simulink library "ddm"  (R2021b)
settings: Solver=VariableStepAuto  StartTime=0.0  StopTime=10.0  RelTol=1e-3
undefined symbols (not defined in the file): ADDM_FrTMTqDev_X_Nm, ADDM_RrTMTqDev_X_Nm, ENUM_ADASACCSTA_ERROR, ENUM_ADASACCSTA_OFF, ENUM_ADASACCSTA_STANDBY, ENUM_ALLOWMOV_ALLOWREADY, ENUM_APS, ENUM_BRKSTA_ERROR, ENUM_BRKSTA_OFF, ENUM_BRKSTA_ON, ENUM_BRKSW_INVALID, ENUM_BRKSW_OFF, ENUM_BRKSW_ON, ENUM_CHGPREACTERRSTA_OBCPRE, ENUM_DCDCFAULTSTA_ANYFAULTLV1, ENUM_DCDCFAULTSTA_ANYFAULTLV2, ENUM_DRIVETRAIN_AWD, ENUM_DRIVETRAIN_FWD, ENUM_DRIVETRAIN_RWD, ENUM_EDUDRTSTA_NORMAL, ENUM_EPBERROR_FAILED, ENUM_EPBSTA_APPLIED, ENUM_EPBSTA_RELEASED, ENUM_ESCAPSSta_APSUNAVAILABLE, ENUM_GEARACTUALPOSN_INVALID, ENUM_GEARACTUALPOSN_P, ENUM_HVBATTREADYPRE_READY, ENUM_HWRESETSTA_HWRESETING, ENUM_MCUWARN_LV0, ENUM_MCUWARN_LV1, ENUM_MCUWARN_LV2, ENUM_MCUWARN_LV3, ENUM_MCUWARN_NOERROR, ENUM_OBCFAULTSTA_ANYFAULT, ENUM_PAS_R2F2, ENUM_PDFAULT_BATTPDFAIL, ENUM_PDFAULT_DCDCDISABLE, ENUM_PDFAULT_MCUDISABLE, ENUM_PDFAULT_MCUDISCHRG, ENUM_POWERSTA_OFF, ENUM_POWERSTA_ON, ENUM_POWERSTA_READY, ENUM_POWERSTA_STANDBY, ENUM_PRESSINDI_LOW, ENUM_PUFAULT_BATTUPFAIL, ENUM_PUFAULT_DCDCENABLEFAIL, ENUM_PUFAULT_PRECHRGCHKFAIL, ENUM_PUFAULT_SAFETYCHKFAIL, ENUM_PWRSTASW_OFF, ENUM_PWRSTASW_OFFA, ENUM_PWRSTASW_OFFCHVCHRG, ENUM_PWRSTASW_OFFCLVCHRG, ENUM_PWRSTASW_ON, ENUM_PWRSTASW_ONHVCHRG, ENUM_PWRSTASW_READY, ENUM_PWRSTASW_STANDBY, ENUM_RAPSErrWarnSta_NORMAL, ENUM_RAPSErrWarnSta_RAPSERRLV1, ENUM_SHIFTCOMMAND_P, ENUM_SHIFTERERRSTA_PBUTTONFAILURE ... (+471)
libraries: hcu_lib x540, simulink x3
(part 12 of 26)

== system ddm/DDM/DDM/TPM/RRBatwarn ==
  note: Diagnostics and Fault Handling
  note: Release Condition After Decision
  note: Test Pass Criteria
  note: Test Detection Criteria
  task_time_s : Inport
  VPMM_PowerSta_enum : Inport  Port=2
  DTC_clear_request : Inport  Port=3
  VTPM_RRBatwarn_flg : Inport  Port=4
  Constant : Constant  Value=KDDM_RRBatwarnDTC_cnt
  Constant1 : Constant  Value=KDDM_RRBatwarnDTC_cnt
  Constant10 : Constant  Value=ENUM_POWERSTA_OFF
  Constant11 : Constant  Value=KDDM_RRBatwarnPassSW_flg
  Constant12 : Constant  Value=FALSE
  Constant13 : Constant  Value=KDDM_RRBatwarnCFSSW_flg
  Constant14 : Constant  Value=KDDM_RRBatwarnDFSSW_flg
  Constant15 : Constant  Value=KDDM_RRBatwarnDetTO_s
  Constant16 : Constant  Value=KDDM_RRBatwarnDetTO_s
  Constant2 : Constant  Value=ENUM_POWERSTA_READY
  Constant24 : Constant  Value=TRUE
  Constant25 : Constant  Value=FALSE
  Constant3 : Constant  Value=ENUM_POWERSTA_ON
  Constant4 : Constant  Value=FALSE
  Constant46 : Constant  Value=KDDM_RRBatwarnDetSW_flg
  Constant5 : Constant  Value=ENUM_POWERSTA_READY
  Constant6 : Constant  Value=KDDM_RRBatwarnDetTO_s
  Constant7 : Constant  Value=ENUM_POWERSTA_ON
  Constant8 : Constant  Value=TRUE
  DTC_Couter : hcu_lib/Basic_Blocks/DTC_Couter
  DTC_Info : hcu_lib/Basic_Blocks/DTC_Info
  Data Type Conversion1 : DataTypeConversion  OutDataTypeStr=uint8
  Equal{1..5} (5 alike) : RelationalOperator  Operator===  OutDataTypeStr=boolean  RndMeth=Simplest
  Equal6 : RelationalOperator  OutDataTypeStr=boolean  RndMeth=Simplest
  Logical Operator1 : Logic  Operator=OR  AllPortsSameDT=off  OutDataTypeStr=boolean
  Logical Operator12 : Logic  AllPortsSameDT=off  OutDataTypeStr=boolean
  Logical Operator15 : Logic  AllPortsSameDT=off  OutDataTypeStr=boolean
  Logical Operator18 : Logic  AllPortsSameDT=off  OutDataTypeStr=boolean
  Logical Operator19 : Logic  Inputs=3  AllPortsSameDT=off  OutDataTypeStr=boolean
  Logical Operator2 : Logic  Operator=NOT  AllPortsSameDT=off  OutDataTypeStr=boolean
  Logical Operator3 : Logic  Operator=OR  Inputs=3  AllPortsSameDT=off  OutDataTypeStr=boolean
  Logical Operator4 : Logic  Operator=OR  AllPortsSameDT=off  OutDataTypeStr=boolean
  Logical Operator5 : Logic  Operator=OR  Inputs=2.  AllPortsSameDT=off  OutDataTypeStr=boolean
  Logical Operator6 : Logic  Operator=NOT  AllPortsSameDT=off  OutDataTypeStr=boolean
  Logical Operator7 : Logic  Operator=OR  Inputs=2.  AllPortsSameDT=off  OutDataTypeStr=boolean
  Logical Operator8 : Logic  Operator=OR  AllPortsSameDT=off  OutDataTypeStr=boolean
  Relay : Relay  OnSwitchValue=ONE_INT  OffSwitchValue=ZERO_INT
  SR_Latch1 : Subsystem  mask(SR_Latch){}
      mask help: SR latch function.
  SR_Latch3 : hcu_lib/Basic_Blocks/SR_Latch
  SR_Latch4 : hcu_lib/Basic_Blocks/SR_Latch
  Switch{2..4,6} (4 alike) : Switch  Criteria=u2 ~= 0
  Test Detection Criteria : hcu_lib/Basic_Blocks/Test Detection Criteria
  Timer1 : hcu_lib/Basic_Blocks/Timer
  VDDM_RRBatwarnDTC_raw32 : Outport
  wires:
  Switch6/1 -> Test Detection Criteria/1
  Constant12/1 -> Switch6/1
  [DTC_clear_request] -> Switch6/2
  Switch3/1 -> [VDDM_RRBatwarnChk_flg], Switch6/3
  VTPM_RRBatwarn_flg/1 -> [VTPM_RRBatwarn_flg]
  [VTPM_RRBatwarn_flg] -> Switch4/1
  Logical Operator4/1 -> Switch4/2
  Equal3/1 -> Logical Operator4/1
  [VPMM_PowerSta_enum] -> Equal2/1
  Constant7/1 -> Equal3/2
  Constant5/1 -> Equal2/2
  Constant8/1 -> Switch4/3
  Equal2/1 -> Logical Operator4/2
  [VPMM_PowerSta_enum] -> Equal3/1
  [VTPM_RRBatwarn_flg] -> Switch3/1
  [task_time_s] -> Test Detection Criteria/2
  Constant/1 -> Test Detection Criteria/3
  Constant6/1 -> Test Detection Criteria/4
  [VPMM_PowerSta_enum] -> Equal5/1
  Equal1/1 -> Logical Operator1/2
  Equal5/1 -> Logical Operator1/1
  Logical Operator1/1 -> Switch3/2
  Constant3/1 -> Equal5/2
  Constant2/1 -> Equal1/2
  Constant4/1 -> Switch3/3
  [VPMM_PowerSta_enum] -> Equal1/1
  [DTC_clear_request] -> DTC_Info/4
  [VDDM_RRBatwarnPass_flg] -> DTC_Info/2
  [VDDM_RRBatwarnDet_flg] -> DTC_Info/1
  Test Detection Criteria/1 -> [VDDM_RRBatwarnDet_flg]  "VDDM_RRBatwarnDet_flg"
  DTC_Info/1 -> VDDM_RRBatwarnDTC_raw32/1  "VDDM_RRBatwarnDTC_raw32"
  [VDDM_RRBatwarnCFS_flg] -> DTC_Info/3
  [VPMM_PowerSta_enum] -> Equal4/1
  DTC_clear_request/1 -> [DTC_clear_request]
  [VDDM_RRBatwarnCFSRls_flg] -> Logical Operator3/3
  Logical Operator18/1 -> [VDDM_RRBatwarnCFS_flg]
  Constant14/1 -> Logical Operator12/1
  SR_Latch3/1 -> Logical Operator12/2
  Constant13/1 -> Logical Operator18/2
  Logical Operator12/1 -> [VDDM_RRBatwarnDFS_flg]
  SR_Latch4/1 -> Logical Operator18/1
  [VDDM_RRBatwarnCFSRls_flg] -> Logical Operator5/1
  [VDDM_RRBatwarnPass_flg] -> Logical Operator3/2
  DTC_Couter/1 -> SR_Latch4/1
  Data Type Conversion1/1 -> [VDDM_RRBatwarnDTC_cnt]  "VDDM_RRBatwarnDTC_cnt"
  Constant46/1 -> Logical Operator19/2
  Logical Operator19/1 -> DTC_Couter/1
  Constant11/1 -> Logical Operator15/2
  Logical Operator15/1 -> DTC_Couter/2
  Constant1/1 -> DTC_Couter/3
  DTC_Couter/2 -> Data Type Conversion1/1
  Relay/1 -> SR_Latch3/1
  [VDDM_RRBatwarnDet_flg] -> Logical Operator19/1
  Logical Operator3/1 -> Logical Operator15/1
  [VDDM_RRBatwarnCFS_flg] -> Logical Operator7/1
  [VDDM_RRBatwarnDTC_cnt] -> Relay/1
  Equal4/1 -> Logical Operator8/1
  Constant10/1 -> Equal4/2
  Constant24/1 -> Switch2/1
  [DTC_clear_request] -> Logical Operator8/2
  Switch2/1 -> [VDDM_RRBatwarnCFSRls_flg]
  Constant25/1 -> Switch2/3
  Logical Operator8/1 -> Switch2/2
  VPMM_PowerSta_enum/1 -> [VPMM_PowerSta_enum]
  task_time_s/1 -> [task_time_s]
  Switch4/1 -> Timer1/2, Logical Operator6/1
  Equal6/1 -> SR_Latch1/1(set)
  [VDDM_RRBatwarnChk_flg] -> SR_Latch1/2(reset)
  Timer1/1 -> Equal6/1
  Constant16/1 -> Equal6/2
  SR_Latch1/1(latched) -> [VDDM_RRBatwarnPass_flg]
  [task_time_s] -> Timer1/3
  Logical Operator6/1 -> Timer1/1
  Constant15/1 -> Timer1/4
  Logical Operator2/1 -> Logical Operator19/3
  [DTC_clear_request] -> Logical Operator3/1, Logical Operator2/1
  Logical Operator5/1 -> SR_Latch4/2
  [DTC_clear_request] -> Logical Operator5/2
  Logical Operator7/1 -> SR_Latch3/2
  [DTC_clear_request] -> Logical Operator7/2

== system ddm/DDM/DDM/TPM/RRPressureLow ==
  note: Test Detection Criteria
  note: Test Pass Criteria
  note: Release Condition After Decision
  note: Diagnostics and Fault Handling
  task_time_s : Inport
  VPMM_PowerSta_enum : Inport  Port=2
  DTC_clear_request : Inport  Port=3
  VTPM_RRPressIndi_enum : Inport  Port=4
  Constant : Constant  Value=KDDM_RRPressIndiDTC_cnt
  Constant1 : Constant  Value=KDDM_RRPressIndiDTC_cnt
  Constant10 : Constant  Value=ENUM_POWERSTA_OFF
  Constant11 : Constant  Value=KDDM_RRPressIndiPassSW_flg
  Constant12 : Constant  Value=FALSE
  Constant13 : Constant  Value=KDDM_RRPressIndiCFSSW_flg
  Constant14 : Constant  Value=KDDM_RRPressIndiDFSSW_flg
  Constant15 : Constant  Value=KDDM_RRPressIndiPassTO_s
  Constant16 : Constant  Value=ENUM_PRESSINDI_LOW
  Constant17 : Constant  Value=ENUM_PRESSINDI_LOW
  Constant2 : Constant  Value=ENUM_POWERSTA_READY
  Constant24 : Constant  Value=TRUE
  Constant25 : Constant  Value=FALSE
  Constant3 : Constant  Value=ENUM_POWERSTA_ON
  Constant4 : Constant  Value=FALSE
  Constant46 : Constant  Value=KDDM_RRPressIndiDetSW_flg
  Constant5 : Constant  Value=ENUM_POWERSTA_READY
  Constant6 : Constant  Value=KDDM_RRPressIndiDetTO_s
  Constant7 : Constant  Value=ENUM_POWERSTA_ON
  Constant8 : Constant  Value=TRUE
  Constant9 : Constant  Value=KDDM_RRPressIndiPassTO_s
  DTC_Couter : hcu_lib/Basic_Blocks/DTC_Couter
  DTC_Info : hcu_lib/Basic_Blocks/DTC_Info
  Data Type Conversion1 : DataTypeConversion  OutDataTypeStr=uint8
  Equal{1..5,7..8} (7 alike) : RelationalOperator  Operator===  OutDataTypeStr=boolean  RndMeth=Simplest
  Equal6 : RelationalOperator  OutDataTypeStr=boolean  RndMeth=Simplest
  Logical Operator{1,4..5,7..8} (5 alike) : Logic  Operator=OR  AllPortsSameDT=off  OutDataTypeStr=boolean
  Logical Operator12 : Logic  AllPortsSameDT=off  OutDataTypeStr=boolean
  Logical Operator15 : Logic  AllPortsSameDT=off  OutDataTypeStr=boolean
  Logical Operator18 : Logic  AllPortsSameDT=off  OutDataTypeStr=boolean
  Logical Operator19 : Logic  Inputs=3  AllPortsSameDT=off  OutDataTypeStr=boolean
  Logical Operator2 : Logic  Operator=NOT  AllPortsSameDT=off  OutDataTypeStr=boolean
  Logical Operator3 : Logic  Operator=OR  Inputs=3  AllPortsSameDT=off  OutDataTypeStr=boolean
  Logical Operator6 : Logic  Operator=NOT  AllPortsSameDT=off  OutDataTypeStr=boolean
  Relay : Relay  OnSwitchValue=ONE_INT  OffSwitchValue=ZERO_INT
  SR_Latch1 : Subsystem  mask(SR_Latch){}
      mask help: SR latch function.
  SR_Latch3 : hcu_lib/Basic_Blocks/SR_Latch
  SR_Latch4 : hcu_lib/Basic_Blocks/SR_Latch
  Switch{2..4,6} (4 alike) : Switch  Criteria=u2 ~= 0
  Test Detection Criteria : hcu_lib/Basic_Blocks/Test Detection Criteria
  Timer1 : hcu_lib/Basic_Blocks/Timer
  VDDM_RRPressIndiDTC_raw32 : Outport
  wires:
  [VTPM_RRPressIndi_enum] -> Equal8/1
  Constant17/1 -> Equal8/2
  Equal8/1 -> Switch4/1
  Constant16/1 -> Equal7/2
  Equal7/1 -> Switch3/1
  [VTPM_RRPressIndi_enum] -> Equal7/1
  task_time_s/1 -> [task_time_s]
  VPMM_PowerSta_enum/1 -> [VPMM_PowerSta_enum]
  Logical Operator8/1 -> Switch2/2
  Constant25/1 -> Switch2/3
  Switch2/1 -> [VDDM_RRPressIndiCFSRls_flg]
  [DTC_clear_request] -> Logical Operator8/2
  Constant24/1 -> Switch2/1
  Constant10/1 -> Equal4/2
  Equal4/1 -> Logical Operator8/1
  [VDDM_RRPressIndiDTC_cnt] -> Relay/1
  [VDDM_RRPressIndiCFS_flg] -> Logical Operator7/1
  Logical Operator3/1 -> Logical Operator15/1
  [VDDM_RRPressIndiDet_flg] -> Logical Operator19/1
  Relay/1 -> SR_Latch3/1
  Constant1/1 -> DTC_Couter/3
  Logical Operator15/1 -> DTC_Couter/2
  Constant11/1 -> Logical Operator15/2
  Logical Operator19/1 -> DTC_Couter/1
  Constant46/1 -> Logical Operator19/2
  DTC_Couter/1 -> SR_Latch4/1
  [VDDM_RRPressIndiPass_flg] -> Logical Operator3/2
  [VDDM_RRPressIndiCFSRls_flg] -> Logical Operator5/1
  SR_Latch4/1 -> Logical Operator18/1
  Logical Operator12/1 -> [VDDM_RRPressIndiDFS_flg]
  Constant13/1 -> Logical Operator18/2
  SR_Latch3/1 -> Logical Operator12/2
  Constant14/1 -> Logical Operator12/1
  Logical Operator18/1 -> [VDDM_RRPressIndiCFS_flg]
  [VDDM_RRPressIndiCFSRls_flg] -> Logical Operator3/3
  DTC_clear_request/1 -> [DTC_clear_request]
  [VPMM_PowerSta_enum] -> Equal4/1
  [VDDM_RRPressIndiCFS_flg] -> DTC_Info/3
  DTC_Info/1 -> VDDM_RRPressIndiDTC_raw32/1  "VDDM_RRPressIndiDTC_raw32"
  Test Detection Criteria/1 -> [VDDM_RRPressIndiDet_flg]  "VDDM_RRPressIndiDet_flg"
  [VDDM_RRPressIndiDet_flg] -> DTC_Info/1
  [VDDM_RRPressIndiPass_flg] -> DTC_Info/2
  [DTC_clear_request] -> DTC_Info/4
  [VPMM_PowerSta_enum] -> Equal1/1
  Constant4/1 -> Switch3/3
  Constant5/1 -> Equal1/2
  Constant7/1 -> Equal5/2
  Logical Operator1/1 -> Switch3/2
  Equal5/1 -> Logical Operator1/1
  Equal1/1 -> Logical Operator1/2
  [VPMM_PowerSta_enum] -> Equal5/1
  Constant6/1 -> Test Detection Criteria/4
  Constant/1 -> Test Detection Criteria/3
  [task_time_s] -> Test Detection Criteria/2
  [VPMM_PowerSta_enum] -> Equal3/1
  Equal2/1 -> Logical Operator4/2
  Constant8/1 -> Switch4/3
  Constant2/1 -> Equal2/2
  Constant3/1 -> Equal3/2
  [VPMM_PowerSta_enum] -> Equal2/1
  Equal3/1 -> Logical Operator4/1
  Logical Operator4/1 -> Switch4/2
  VTPM_RRPressIndi_enum/1 -> [VTPM_RRPressIndi_enum]
  Switch3/1 -> [VDDM_RRPressIndiChk_flg], Switch6/3
  [DTC_clear_request] -> Switch6/2
  Constant12/1 -> Switch6/1
  Switch6/1 -> Test Detection Criteria/1
  Switch4/1 -> Logical Operator6/1, Timer1/2
  Equal6/1 -> SR_Latch1/1(set)
  Constant9/1 -> Equal6/2
  SR_Latch1/1(latched) -> [VDDM_RRPressIndiPass_flg]
  [VDDM_RRPressIndiChk_flg] -> SR_Latch1/2(reset)
  [task_time_s] -> Timer1/3
  Timer1/1 -> Equal6/1
  Constant15/1 -> Timer1/4
  Logical Operator6/1 -> Timer1/1
  Data Type Conversion1/1 -> [VDDM_RRPressIndiDTC_cnt]  "VDDM_RRPressIndiDTC_cnt"
  DTC_Couter/2 -> Data Type Conversion1/1
  Logical Operator2/1 -> Logical Operator19/3
  [DTC_clear_request] -> Logical Operator3/1, Logical Operator2/1
  Logical Operator5/1 -> SR_Latch4/2
  [DTC_clear_request] -> Logical Operator5/2
  Logical Operator7/1 -> SR_Latch3/2
  [DTC_clear_request] -> Logical Operator7/2

== system ddm/DDM/DDM/TPM/RRSensorfail ==
  note: Test Detection Criteria
  note: Test Pass Criteria
  note: Release Condition After Decision
  note: Diagnostics and Fault Handling
  task_time_s : Inport
  VPMM_PowerSta_enum : Inport  Port=2
  DTC_clear_request : Inport  Port=3
  VTPM_RRSensorFail_flg : Inport  Port=4
  Constant : Constant  Value=KDDM_RRSensorFailDTC_cnt
  Constant1 : Constant  Value=KDDM_RRSensorFailDTC_cnt
  Constant10 : Constant  Value=ENUM_POWERSTA_OFF
  Constant11 : Constant  Value=KDDM_RRSensorFailPassSW_flg
  Constant12 : Constant  Value=FALSE
  Constant13 : Constant  Value=KDDM_RRSensorFailCFSSW_flg
  Constant14 : Constant  Value=KDDM_RRSensorFailDFSSW_flg
  Constant15 : Constant  Value=KDDM_RRSensorFailPassTO_s
  Constant2 : Constant  Value=ENUM_POWERSTA_READY
  Constant24 : Constant  Value=TRUE
  Constant25 : Constant  Value=FALSE
  Constant3 : Constant  Value=ENUM_POWERSTA_ON
  Constant4 : Constant  Value=FALSE
  Constant46 : Constant  Value=KDDM_RRSensorFailDetSW_flg
  Constant5 : Constant  Value=ENUM_POWERSTA_READY
  Constant6 : Constant  Value=KDDM_RRSensorFailDetTO_s
  Constant7 : Constant  Value=ENUM_POWERSTA_ON
  Constant8 : Constant  Value=TRUE
  Constant9 : Constant  Value=KDDM_RRSensorFailPassTO_s
  DTC_Couter : hcu_lib/Basic_Blocks/DTC_Couter
  DTC_Info : hcu_lib/Basic_Blocks/DTC_Info
  Data Type Conversion1 : DataTypeConversion  OutDataTypeStr=uint8
  Equal{1..5} (5 alike) : RelationalOperator  Operator===  OutDataTypeStr=boolean  RndMeth=Simplest
  Equal6 : RelationalOperator  OutDataTypeStr=boolean  RndMeth=Simplest
  Logical Operator{1..2,4,7..8} (5 alike) : Logic  Operator=OR  AllPortsSameDT=off  OutDataTypeStr=boolean
  Logical Operator12 : Logic  AllPortsSameDT=off  OutDataTypeStr=boolean
  Logical Operator15 : Logic  AllPortsSameDT=off  OutDataTypeStr=boolean
  Logical Operator18 : Logic  AllPortsSameDT=off  OutDataTypeStr=boolean
  Logical Operator19 : Logic  Inputs=3  AllPortsSameDT=off  OutDataTypeStr=boolean
  Logical Operator3 : Logic  Operator=OR  Inputs=3  AllPortsSameDT=off  OutDataTypeStr=boolean
  Logical Operator5 : Logic  Operator=NOT  AllPortsSameDT=off  OutDataTypeStr=boolean
  Logical Operator6 : Logic  Operator=NOT  AllPortsSameDT=off  OutDataTypeStr=boolean
  Relay : Relay  OnSwitchValue=ONE_INT  OffSwitchValue=ZERO_INT
  SR_Latch1 : Subsystem  mask(SR_Latch){}
      mask help: SR latch function.
  SR_Latch3 : hcu_lib/Basic_Blocks/SR_Latch
  SR_Latch4 : hcu_lib/Basic_Blocks/SR_Latch
  Switch{2..4,6} (4 alike) : Switch  Criteria=u2 ~= 0
  Test Detection Criteria : hcu_lib/Basic_Blocks/Test Detection Criteria
  Timer1 : hcu_lib/Basic_Blocks/Timer
  VDDM_RRSensorFailDTC_raw32 : Outport
  wires:
  [VTPM_RRSensorFail_flg] -> Switch4/1
  [VTPM_RRSensorFail_flg] -> Switch3/1
  task_time_s/1 -> [task_time_s]
  VPMM_PowerSta_enum/1 -> [VPMM_PowerSta_enum]
  Logical Operator8/1 -> Switch2/2
  Constant25/1 -> Switch2/3
  Switch2/1 -> [VDDM_RRSensorFailCFSRls_flg]
  [DTC_clear_request] -> Logical Operator8/2
  Constant24/1 -> Switch2/1
  Constant10/1 -> Equal4/2
  Equal4/1 -> Logical Operator8/1
  [VDDM_RRSensorFailDTC_cnt] -> Relay/1
  [VDDM_RRSensorFailCFS_flg] -> Logical Operator7/1
  Logical Operator3/1 -> Logical Operator15/1
  [VDDM_RRSensorFailDet_flg] -> Logical Operator19/1
  Relay/1 -> SR_Latch3/1
  DTC_Couter/2 -> Data Type Conversion1/1
  Constant1/1 -> DTC_Couter/3
  Logical Operator15/1 -> DTC_Couter/2
  Constant11/1 -> Logical Operator15/2
  Logical Operator19/1 -> DTC_Couter/1
  Constant46/1 -> Logical Operator19/2
  Data Type Conversion1/1 -> [VDDM_RRSensorFailDTC_cnt]  "VDDM_RRSensorFailDTC_cnt"
  DTC_Couter/1 -> SR_Latch4/1
  [VDDM_RRSensorFailPass_flg] -> Logical Operator3/2
  [VDDM_RRSensorFailCFSRls_flg] -> Logical Operator2/1
  SR_Latch4/1 -> Logical Operator18/1
  Logical Operator12/1 -> [VDDM_RRSensorFailDFS_flg]
  Constant13/1 -> Logical Operator18/2
  SR_Latch3/1 -> Logical Operator12/2
  Constant14/1 -> Logical Operator12/1
  Logical Operator18/1 -> [VDDM_RRSensorFailCFS_flg]
  [VDDM_RRSensorFailCFSRls_flg] -> Logical Operator3/3
  DTC_clear_request/1 -> [DTC_clear_request]
  [VPMM_PowerSta_enum] -> Equal4/1
  [VDDM_RRSensorFailCFS_flg] -> DTC_Info/3
  DTC_Info/1 -> VDDM_RRSensorFailDTC_raw32/1  "VDDM_RRSensorFailDTC_raw32"
  Test Detection Criteria/1 -> [VDDM_RRSensorFailDet_flg]  "VDDM_RRSensorFailDet_flg"
  [VDDM_RRSensorFailDet_flg] -> DTC_Info/1
  [VDDM_RRSensorFailPass_flg] -> DTC_Info/2
  [DTC_clear_request] -> DTC_Info/4
  [VPMM_PowerSta_enum] -> Equal1/1
  Constant4/1 -> Switch3/3
  Constant5/1 -> Equal1/2
  Constant7/1 -> Equal5/2
  Logical Operator1/1 -> Switch3/2
  Equal5/1 -> Logical Operator1/1
  Equal1/1 -> Logical Operator1/2
  [VPMM_PowerSta_enum] -> Equal5/1
  Constant6/1 -> Test Detection Criteria/4
  Constant/1 -> Test Detection Criteria/3
  [task_time_s] -> Test Detection Criteria/2
  [VPMM_PowerSta_enum] -> Equal3/1
  Equal2/1 -> Logical Operator4/2
  Constant8/1 -> Switch4/3
  Constant2/1 -> Equal2/2
  Constant3/1 -> Equal3/2
  [VPMM_PowerSta_enum] -> Equal2/1
  Equal3/1 -> Logical Operator4/1
  Logical Operator4/1 -> Switch4/2
  VTPM_RRSensorFail_flg/1 -> [VTPM_RRSensorFail_flg]
  Switch3/1 -> [VDDM_RRSensorFailChk_flg], Switch6/3
  [DTC_clear_request] -> Switch6/2
  Constant12/1 -> Switch6/1
  Switch6/1 -> Test Detection Criteria/1
  Switch4/1 -> Timer1/2, Logical Operator6/1
  Equal6/1 -> SR_Latch1/1(set)
  Constant9/1 -> Equal6/2
  SR_Latch1/1(latched) -> [VDDM_RRSensorFailPass_flg]
  [VDDM_RRSensorFailChk_flg] -> SR_Latch1/2(reset)
  [task_time_s] -> Timer1/3
  Timer1/1 -> Equal6/1
  Constant15/1 -> Timer1/4
  Logical Operator6/1 -> Timer1/1
  Logical Operator5/1 -> Logical Operator19/3
  [DTC_clear_request] -> Logical Operator3/1, Logical Operator5/1
  Logical Operator2/1 -> SR_Latch4/2
  [DTC_clear_request] -> Logical Operator2/2
  Logical Operator7/1 -> SR_Latch3/2
  [DTC_clear_request] -> Logical Operator7/2

== system ddm/DDM/DDM/TPM/RRWheelTmpHigh ==
  note: Diagnostics and Fault Handling
  note: Release Condition After Decision
  note: Test Pass Criteria
  note: Test Detection Criteria
  task_time_s : Inport
  VPMM_PowerSta_enum : Inport  Port=2
  DTC_clear_request : Inport  Port=3
  VTPM_RRWheelTmpHigh_flg : Inport  Port=4
  Constant : Constant  Value=KDDM_RRWheelTmpHighDTC_cnt
  Constant1 : Constant  Value=KDDM_RRWheelTmpHighDTC_cnt
  Constant10 : Constant  Value=ENUM_POWERSTA_OFF
  Constant11 : Constant  Value=KDDM_RRWheelTmpHighPassSW_flg
  Constant12 : Constant  Value=FALSE
  Constant13 : Constant  Value=KDDM_RRWheelTmpHighCFSSW_flg
  Constant14 : Constant  Value=KDDM_RRWheelTmpHighDFSSW_flg
  Constant15 : Constant  Value=KDDM_RRWheelTmpHighPassTO_s
  Constant2 : Constant  Value=ENUM_POWERSTA_READY
  Constant24 : Constant  Value=TRUE
  Constant25 : Constant  Value=FALSE
  Constant3 : Constant  Value=ENUM_POWERSTA_ON
  Constant4 : Constant  Value=FALSE
  Constant46 : Constant  Value=KDDM_RRWheelTmpHighDetSW_flg
  Constant5 : Constant  Value=ENUM_POWERSTA_READY
  Constant6 : Constant  Value=KDDM_RRWheelTmpHighDetTO_s
  Constant7 : Constant  Value=ENUM_POWERSTA_ON
  Constant8 : Constant  Value=TRUE
  Constant9 : Constant  Value=KDDM_RRWheelTmpHighPassTO_s
  DTC_Couter : hcu_lib/Basic_Blocks/DTC_Couter
  DTC_Info : hcu_lib/Basic_Blocks/DTC_Info
  Data Type Conversion1 : DataTypeConversion  OutDataTypeStr=uint8
  Equal{1..5} (5 alike) : RelationalOperator  Operator===  OutDataTypeStr=boolean  RndMeth=Simplest
  Equal6 : RelationalOperator  OutDataTypeStr=boolean  RndMeth=Simplest
  Logical Operator{1..2,4,7..8} (5 alike) : Logic  Operator=OR  AllPortsSameDT=off  OutDataTypeStr=boolean
  Logical Operator12 : Logic  AllPortsSameDT=off  OutDataTypeStr=boolean
  Logical Operator15 : Logic  AllPortsSameDT=off  OutDataTypeStr=boolean
  Logical Operator18 : Logic  AllPortsSameDT=off  OutDataTypeStr=boolean
  Logical Operator19 : Logic  Inputs=3  AllPortsSameDT=off  OutDataTypeStr=boolean
  Logical Operator3 : Logic  Operator=OR  Inputs=3  AllPortsSameDT=off  OutDataTypeStr=boolean
  Logical Operator5 : Logic  Operator=NOT  AllPortsSameDT=off  OutDataTypeStr=boolean
  Logical Operator6 : Logic  Operator=NOT  AllPortsSameDT=off  OutDataTypeStr=boolean
  Relay : Relay  OnSwitchValue=ONE_INT  OffSwitchValue=ZERO_INT
  SR_Latch1 : Subsystem  mask(SR_Latch){}
      mask help: SR latch function.
  SR_Latch3 : hcu_lib/Basic_Blocks/SR_Latch
  SR_Latch4 : hcu_lib/Basic_Blocks/SR_Latch
  Switch{2..4,6} (4 alike) : Switch  Criteria=u2 ~= 0
  Test Detection Criteria : hcu_lib/Basic_Blocks/Test Detection Criteria
  Timer1 : hcu_lib/Basic_Blocks/Timer
  VDDM_RRWheelTmpHighDTC_raw32 : Outport
  wires:
  Logical Operator6/1 -> Timer1/1
  Constant15/1 -> Timer1/4
  Timer1/1 -> Equal6/1
  [task_time_s] -> Timer1/3
  [VDDM_RRWheelTmpHighChk_flg] -> SR_Latch1/2(reset)
  SR_Latch1/1(latched) -> [VDDM_RRWheelTmpHighPass_flg]
  Constant9/1 -> Equal6/2
  Equal6/1 -> SR_Latch1/1(set)
  Switch4/1 -> Logical Operator6/1, Timer1/2
  Switch6/1 -> Test Detection Criteria/1
  Constant12/1 -> Switch6/1
  [DTC_clear_request] -> Switch6/2
  Switch3/1 -> Switch6/3, [VDDM_RRWheelTmpHighChk_flg]
  VTPM_RRWheelTmpHigh_flg/1 -> [VTPM_RRWheelTmpHigh_flg]
  Logical Operator4/1 -> Switch4/2
  Equal3/1 -> Logical Operator4/1
  [VPMM_PowerSta_enum] -> Equal2/1
  Constant3/1 -> Equal3/2
  Constant2/1 -> Equal2/2
  Constant8/1 -> Switch4/3
  Equal2/1 -> Logical Operator4/2
  [VPMM_PowerSta_enum] -> Equal3/1
  [task_time_s] -> Test Detection Criteria/2
  Constant/1 -> Test Detection Criteria/3
  Constant6/1 -> Test Detection Criteria/4
  [VPMM_PowerSta_enum] -> Equal5/1
  Equal1/1 -> Logical Operator1/2
  Equal5/1 -> Logical Operator1/1
  Logical Operator1/1 -> Switch3/2
  Constant7/1 -> Equal5/2
  Constant5/1 -> Equal1/2
  Constant4/1 -> Switch3/3
  [VPMM_PowerSta_enum] -> Equal1/1
  [DTC_clear_request] -> DTC_Info/4
  [VDDM_RRWheelTmpHighPass_flg] -> DTC_Info/2
  [VDDM_RRWheelTmpHighDet_flg] -> DTC_Info/1
  Test Detection Criteria/1 -> [VDDM_RRWheelTmpHighDet_flg]  "VDDM_RRWheelTmpHighDet_flg"
  DTC_Info/1 -> VDDM_RRWheelTmpHighDTC_raw32/1  "VDDM_RRWheelTmpHighDTC_raw32"
  [VDDM_RRWheelTmpHighCFS_flg] -> DTC_Info/3
  [VPMM_PowerSta_enum] -> Equal4/1
  DTC_clear_request/1 -> [DTC_clear_request]
  [VDDM_RRWheelTmpHighCFSRls_flg] -> Logical Operator3/3
  Logical Operator18/1 -> [VDDM_RRWheelTmpHighCFS_flg]
  Constant14/1 -> Logical Operator12/1
  SR_Latch3/1 -> Logical Operator12/2
  Constant13/1 -> Logical Operator18/2
  Logical Operator12/1 -> [VDDM_RRWheelTmpHighDFS_flg]
  SR_Latch4/1 -> Logical Operator18/1
  [VDDM_RRWheelTmpHighCFSRls_flg] -> Logical Operator2/1
  [VDDM_RRWheelTmpHighPass_flg] -> Logical Operator3/2
  DTC_Couter/1 -> SR_Latch4/1
  Data Type Conversion1/1 -> [VDDM_RRWheelTmpHighDTC_cnt]  "VDDM_RRWheelTmpHighDTC_cnt"
  Constant46/1 -> Logical Operator19/2
  Logical Operator19/1 -> DTC_Couter/1
  Constant11/1 -> Logical Operator15/2
  Logical Operator15/1 -> DTC_Couter/2
  Constant1/1 -> DTC_Couter/3
  DTC_Couter/2 -> Data Type Conversion1/1
  Relay/1 -> SR_Latch3/1
  [VDDM_RRWheelTmpHighDet_flg] -> Logical Operator19/1
  Logical Operator3/1 -> Logical Operator15/1
  [VDDM_RRWheelTmpHighCFS_flg] -> Logical Operator7/1
  [VDDM_RRWheelTmpHighDTC_cnt] -> Relay/1
  Equal4/1 -> Logical Operator8/1
  Constant10/1 -> Equal4/2
  Constant24/1 -> Switch2/1
  [DTC_clear_request] -> Logical Operator8/2
  Switch2/1 -> [VDDM_RRWheelTmpHighCFSRls_flg]
  Constant25/1 -> Switch2/3
  Logical Operator8/1 -> Switch2/2
  VPMM_PowerSta_enum/1 -> [VPMM_PowerSta_enum]
  task_time_s/1 -> [task_time_s]
  [VTPM_RRWheelTmpHigh_flg] -> Switch3/1
  [VTPM_RRWheelTmpHigh_flg] -> Switch4/1
  Logical Operator5/1 -> Logical Operator19/3
  [DTC_clear_request] -> Logical Operator3/1, Logical Operator5/1
  Logical Operator2/1 -> SR_Latch4/2
  [DTC_clear_request] -> Logical Operator2/2
  Logical Operator7/1 -> SR_Latch3/2
  [DTC_clear_request] -> Logical Operator7/2

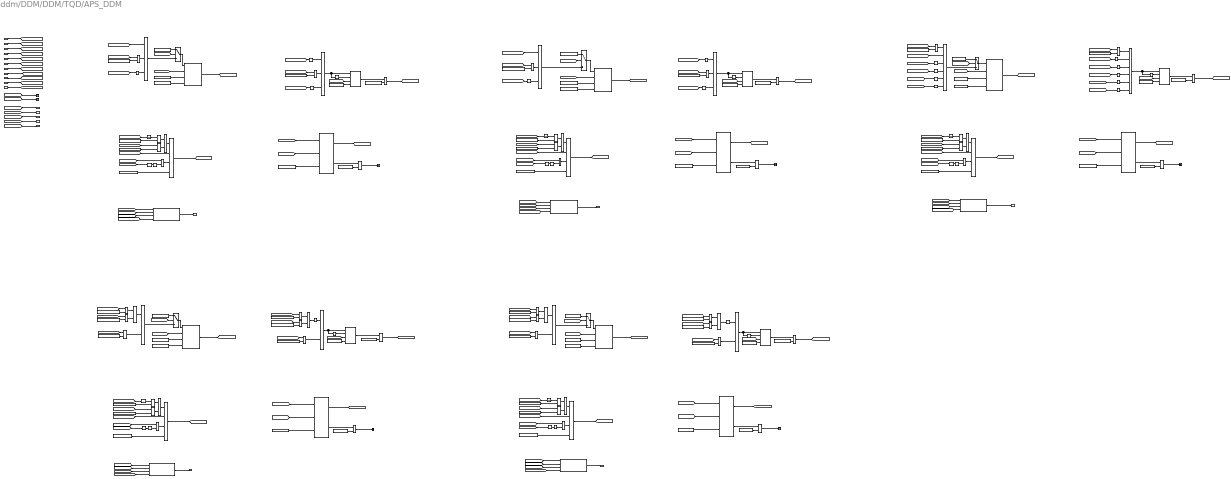
== system ddm/DDM/DDM/TQD/APS_DDM ==
  note: Release Condition After Decision
  note: Diagnostics and Fault Handling
  note: Diagnostics and Fault Handling
  note: Release Condition After Decision
  note: Release Condition After Decision
  note: Diagnostics and Fault Handling
  note: Diagnostics and Fault Handling
  note: Release Condition After Decision
  note: Release Condition After Decision
  note: Diagnostics and Fault Handling
  note: APS1 Signal Out of Range (APS1SigOoR)
  note: APS1 5V Out of Range (5vAPS1OoR)
  note: APS Correlation Error (APSCorrErr)
  note: APS2 Signal Out of Range (APS2SigOoR)
  note: APS2 5V Out of Range (5vAPS2OoR)
  VPMM_SysPwrSta_enum : Inport
  VINP_AccelPedal1Vol_V : Inport  Port=2
  VINP_AccelPedal2Vol_V : Inport  Port=3
  VDHP_EAPS12RangeSta_enum : Inport  Port=4
  VDHP_EAPCRBAD_flg : Inport  Port=5
  VINP_Pedal1Ref5V_V : Inport  Port=6
  VINP_Pedal2Ref5V_V : Inport  Port=7
  task_time_s : Inport  Port=8
  DTC_clear_request : Inport  Port=9
  VDHP_EAPS1BAD_flg : Inport  Port=10
  VDHP_EAPS2BAD_flg : Inport  Port=11
  Constant{1,7,10,14,17,23,27,34..39,41,48} (15 alike) : Constant  Value=ENUM_PWRSTASW_OFF
  Constant107 : Constant  Value=KDDM_APS2SigOoRPassTO_s
  Constant108 : Constant  Value=KDDM_APS2SigOoRPassTO_s
  Constant109 : Constant  Value=KDDM_5vAPS2OoRPassTO_s
  Constant{4,11,24,26,45} (5 alike) : Constant  Value=ENUM_PWRSTASW_STANDBY
  Constant{21,85,90,99,111} (5 alike) : Constant  Value=FALSE
  Constant112 : Constant  Value=KDDM_5vAPS2OoRDetTO_s
  Constant118 : Constant  Value=KDDM_5vAPS2OoRDTC_cnt
  Constant{6,12,31,46,53} (5 alike) : Constant  Value=KDDM_TQDDiagnosisOffSW_flg
  Constant{13,16,32,47,54} (5 alike) : Constant  Value=ZERO_INT
  Constant132 : Constant  Value=KDDM_APS1SigOoRDTC_cnt
  Constant15 : Constant  Value=KDDM_APS2SigOoRDTC_cnt
  Constant18 : Constant  Value=KDDM_5vAPS2OoRDTC_cnt
  Constant19 : Constant  Value=KDDM_5vAPS1OoRPassTO_s
  Constant2 : Constant  Value=KDDM_5vAPS1OoRHiLim_V
  Constant20 : Constant  Value=KDDM_5vAPS1OoRPassTO_s
  Constant22 : Constant  Value=KDDM_5vAPS1OoRDetTO_s
  Constant25 : Constant  Value=KDDM_5vAPS2OoRHiLim_V
  Constant28 : Constant  Value=KDDM_5vAPS2OoRHiLim_V
  Constant29 : Constant  Value=KDDM_5vAPS2OoRLoLim_V
  Constant3 : Constant  Value=KDDM_5vAPS1OoRLoLim_V
  Constant30 : Constant  Value=KDDM_5vAPS2OoRPassTO_s
  Constant33 : Constant  Value=KDDM_5vAPS2OoRLoLim_V
  Constant49 : Constant  Value=KDDM_APS1SigOoRDTC_cnt
  Constant5 : Constant  Value=KDDM_5vAPS1OoRDTC_cnt
  Constant50 : Constant  Value=KDDM_APS2SigOoRDTC_cnt
  Constant55 : Constant  Value=KDDM_APSCorrErrPassTO_s
  Constant57 : Constant  Value=KDDM_APSCorrErrDetTO_s
  Constant58 : Constant  Value=KDDM_APSCorrErrDTC_cnt
  Constant59 : Constant  Value=KDDM_APSCorrErrDTC_cnt
  Constant65 : Constant  Value=KDDM_5vAPS1OoRDTC_cnt
  Constant68 : Constant  Value=KDDM_APS2SigOoRDetTO_s
  Constant69 : Constant  Value=KDDM_APS1SigOoRPassTO_s
  Constant70 : Constant  Value=KDDM_APS1SigOoRPassTO_s
  Constant8 : Constant  Value=KDDM_5vAPS1OoRHiLim_V
  Constant86 : Constant  Value=KDDM_APS1SigOoRDetTO_s
  Constant9 : Constant  Value=KDDM_5vAPS1OoRLoLim_V
  Constant91 : Constant  Value=KDDM_APSCorrErrPassTO_s
  DTC_Couter{1..4,6} (5 alike) : hcu_lib/Basic_Blocks/DTC_Couter
  DTC_Info{,1..4} (5 alike) : hcu_lib/Basic_Blocks/DTC_Info
  Delay{1..5} (5 alike) : Delay  DelayLength=1
  Equal{1,3,6,13,15..16,19,21,26,47} (10 alike) : RelationalOperator  Operator=~=  OutDataTypeStr=boolean  RndMeth=Simplest
  Equal{4,10..12,18,23..25,39..40} (10 alike) : RelationalOperator  Operator===  OutDataTypeStr=boolean  RndMeth=Simplest
  Equal{2,7,14,20} (4 alike) : RelationalOperator  Operator=>  OutDataTypeStr=boolean  RndMeth=Simplest
  Equal{5,8,17,27} (4 alike) : RelationalOperator  Operator=<  OutDataTypeStr=boolean  RndMeth=Simplest
  Equal{9,28,55,65,70} (5 alike) : RelationalOperator  OutDataTypeStr=boolean  RndMeth=Simplest
  Logical Operator{1..2,14,17} (4 alike) : Logic  Operator=OR  AllPortsSameDT=off  OutDataTypeStr=boolean
  Logical Operator{3,7,10..12,19..20,22,29,34,37,39,41..42} (14 alike) : Logic  AllPortsSameDT=off  OutDataTypeStr=boolean
  Logical Operator{4,8,13,15..16,21,23..28,30,32,36,40,44..45,62,73,83,112} (22 alike) : Logic  Operator=NOT  AllPortsSameDT=off  OutDataTypeStr=boolean
  Logical Operator{6,9,18,38,43} (5 alike) : Logic  Operator=OR  Inputs=4  AllPortsSameDT=off  OutDataTypeStr=boolean
  Logical Operator{5,31,33,35} (4 alike) : Logic  Inputs=3  AllPortsSameDT=off  OutDataTypeStr=boolean
  Logical Operator49 : Logic  Inputs=6  AllPortsSameDT=off  OutDataTypeStr=boolean
  Logical Operator86 : Logic  Inputs=6  AllPortsSameDT=off  OutDataTypeStr=boolean
  NOT{1..5} (5 alike) : Logic  Operator=NOT  AllPortsSameDT=off  OutDataTypeStr=boolean
  Relational Operator{1..5} (5 alike) : RelationalOperator  Operator=>  OutDataTypeStr=boolean  RndMeth=Simplest
  Switch{1..4,6} (5 alike) : Switch  Criteria=u2 ~= 0
  Terminator{,1..6} (7 alike) : Terminator
  Test Detection Criteria{1..5} (5 alike) : hcu_lib/Basic_Blocks/Test Detection Criteria
  Timer{1,4..5,13,15} (5 alike) : hcu_lib/Basic_Blocks/Timer
  Unit Delay{1,3..6} (5 alike) : UnitDelay  SampleTime=-1  HasFrameUpgradeWarning=on
  VDDM_APS1SigOoRDTC_raw32 : Outport
  VDDM_APS2SigOoRDTC_raw32 : Outport  Port=2
  VDDM_APSCorrErrDTC_raw32 : Outport  Port=3
  VDDM_5vAPS1OoRDTC_raw32 : Outport  Port=4
  VDDM_5vAPS2OoRDTC_raw32 : Outport  Port=5
  VDDM_5vAPS1OoRCFS_flg : Outport  Port=6
  VDDM_5vAPS2OoRCFS_flg : Outport  Port=7
  VDDM_APS1SigOoRCFS_flg : Outport  Port=8
  VDDM_APS2SigOoRCFS_flg : Outport  Port=9
  VDDM_APSCorrErrCFS_flg : Outport  Port=10
  wires:
  Logical Operator44/1 -> Logical Operator49/6
  Logical Operator27/1 -> Logical Operator49/5
  Logical Operator26/1 -> Logical Operator49/4
  Logical Operator25/1 -> Logical Operator49/3
  Logical Operator24/1 -> Logical Operator86/6
  Logical Operator21/1 -> Logical Operator86/5
  Logical Operator16/1 -> Logical Operator86/4
  Logical Operator15/1 -> Logical Operator86/3
  Logical Operator13/1 -> Logical Operator35/1
  [VDDM_APS1SigOoRCFS_flg] -> Logical Operator27/1
  [VDDM_APS2SigOoRCFS_flg] -> Logical Operator44/1
  [VDDM_5vAPS2OoRCFS_flg] -> Logical Operator26/1
  [VDDM_5vAPS1OoRCFS_flg] -> Logical Operator25/1
  Equal26/1 -> Logical Operator49/1
  Constant41/1 -> Equal26/2
  [VPMM_SysPwrSta_enum] -> Equal26/1
  [VDDM_APS2SigOoRCFS_flg] -> Logical Operator24/1
  [VDDM_APS1SigOoRCFS_flg] -> Logical Operator21/1
  [VDDM_5vAPS2OoRCFS_flg] -> Logical Operator16/1
  [VDDM_5vAPS1OoRCFS_flg] -> Logical Operator15/1
  Equal21/1 -> Logical Operator86/1
  [VPMM_SysPwrSta_enum] -> Equal21/1
  Constant39/1 -> Equal21/2
  [VPMM_SysPwrSta_enum] -> Equal16/1
  Constant38/1 -> Equal16/2
  [VPMM_SysPwrSta_enum] -> Equal3/1
  Constant10/1 -> Equal3/2
  [VPMM_SysPwrSta_enum] -> Equal15/1
  Constant37/1 -> Equal15/2
  [VPMM_SysPwrSta_enum] -> Equal47/1
  Constant36/1 -> Equal47/2
  [VDDM_APSCorrErrCFS_flg] -> VDDM_APSCorrErrCFS_flg/1
  [VDDM_APS2SigOoRCFS_flg] -> VDDM_APS2SigOoRCFS_flg/1
  [VDDM_APS1SigOoRCFS_flg] -> VDDM_APS1SigOoRCFS_flg/1
  [VDDM_5vAPS2OoRCFS_flg] -> VDDM_5vAPS2OoRCFS_flg/1
  [VDDM_5vAPS1OoRCFS_flg] -> VDDM_5vAPS1OoRCFS_flg/1
  Logical Operator23/1 -> Logical Operator22/1
  Equal27/1 -> Logical Operator14/2
  Constant29/1 -> Equal27/2
  Equal20/1 -> Logical Operator14/1
  [VINP_Pedal2Ref5V_V] -> Equal20/1
  Logical Operator14/1 -> Logical Operator23/1
  Constant28/1 -> Equal20/2
  Constant27/1 -> Equal19/2
  [VPMM_SysPwrSta_enum] -> Equal19/1
  [VINP_Pedal2Ref5V_V] -> Equal27/1
  Equal19/1 -> Logical Operator22/2
  Equal13/1 -> Logical Operator20/2
  [VINP_Pedal2Ref5V_V] -> Equal17/1
  [VPMM_SysPwrSta_enum] -> Equal13/1
  Constant23/1 -> Equal13/2
  Constant25/1 -> Equal14/2
  Logical Operator17/1 -> Logical Operator20/1
  [VINP_Pedal2Ref5V_V] -> Equal14/1
  Equal14/1 -> Logical Operator17/1
  Constant33/1 -> Equal17/2
  Equal17/1 -> Logical Operator17/2
  [VDDM_5vAPS2OoRDet_flg] -> DTC_Couter4/1
  [VDDM_5vAPS2OoRCFSRls_flg] -> DTC_Couter4/2
  [VPMM_SysPwrSta_enum] -> Unit Delay1/1
  Constant16/1 -> Relational Operator5/2
  [VDDM_5vAPS2OoRCFS_flg] -> Delay5/1
  Logical Operator10/1 -> Logical Operator9/1
  Equal11/1 -> Logical Operator10/1
  Constant6/1 -> Logical Operator9/4
  Logical Operator9/1 -> [VDDM_5vAPS2OoRCFSRls_flg]  "VDDM_5vAPS2OoRCFSRls_flg"
  Delay5/1 -> NOT5/1
  NOT5/1 -> Logical Operator11/2
  [DTC_clear_request] -> Logical Operator9/2
  Constant4/1 -> Equal10/2
  Constant18/1 -> DTC_Couter4/3
  Equal10/1 -> Logical Operator10/2
  DTC_Couter4/2 -> Relational Operator5/1  "VDDM_5vAPS2OoRDTC_cnt"
  [VPMM_SysPwrSta_enum] -> Equal10/1
  Logical Operator11/1 -> Logical Operator9/3
  Constant17/1 -> Equal11/2
  Unit Delay1/1 -> Equal11/1
  Relational Operator5/1 -> Terminator4/1  "VDDM_5vAPS2OoRDFS_flg"
  [VDDM_5vAPS2OoRPass_flg] -> Logical Operator11/1
  DTC_Couter4/1 -> [VDDM_5vAPS2OoRCFS_flg]  "VDDM_5vAPS2OoRCFS_flg"
  Logical Operator8/1 -> Logical Operator7/1
  Equal6/1 -> Logical Operator7/2
  [VINP_Pedal1Ref5V_V] -> Equal8/1
  [VPMM_SysPwrSta_enum] -> Equal6/1
  Constant1/1 -> Equal6/2
  Constant2/1 -> Equal7/2
  Logical Operator1/1 -> Logical Operator8/1
  [VINP_Pedal1Ref5V_V] -> Equal7/1
  Equal7/1 -> Logical Operator1/1
  Constant3/1 -> Equal8/2
  Equal8/1 -> Logical Operator1/2
  Constant65/1 -> DTC_Couter3/3
  [VDDM_5vAPS1OoRDet_flg] -> DTC_Couter3/1
  Equal12/1 -> Logical Operator19/2
  Relational Operator4/1 -> Terminator3/1  "VDDM_5vAPS1OoRDFS_flg"
  [VDDM_5vAPS1OoRCFSRls_flg] -> DTC_Couter3/2
  [VDDM_5vAPS1OoRPass_flg] -> Logical Operator34/1
  Logical Operator18/1 -> [VDDM_5vAPS1OoRCFSRls_flg]  "VDDM_5vAPS1OoRCFSRls_flg"
  Constant31/1 -> Logical Operator18/4
  Logical Operator19/1 -> Logical Operator18/1
  [VPMM_SysPwrSta_enum] -> Unit Delay5/1
  Constant24/1 -> Equal12/2
  [DTC_clear_request] -> Logical Operator18/2
  NOT4/1 -> Logical Operator34/2
  Delay4/1 -> NOT4/1
  DTC_Couter3/1 -> [VDDM_5vAPS1OoRCFS_flg]  "VDDM_5vAPS1OoRCFS_flg"
  Equal18/1 -> Logical Operator19/1
  Unit Delay5/1 -> Equal18/1
  Constant35/1 -> Equal18/2
  Constant32/1 -> Relational Operator4/2
  DTC_Couter3/2 -> Relational Operator4/1  "VDDM_5vAPS1OoRDTC_cnt"
  Logical Operator34/1 -> Logical Operator18/3
  [VPMM_SysPwrSta_enum] -> Equal12/1
  [VDDM_5vAPS1OoRCFS_flg] -> Delay4/1
  Constant7/1 -> Equal1/2
  [VPMM_SysPwrSta_enum] -> Equal1/1
  Unit Delay4/1 -> Equal39/1
  Constant54/1 -> Relational Operator3/2
  Constant34/1 -> Equal39/2
  DTC_Couter2/2 -> Relational Operator3/1  "VDDM_APSCorrErrDTC_cnt"
  Logical Operator42/1 -> Logical Operator43/3
  [VDDM_APSCorrErrCFS_flg] -> Delay3/1
  Logical Operator43/1 -> [VDDM_APSCorrErrCFSRls_flg]  "VDDM_APSCorrErrCFSRls_flg"
  [VPMM_SysPwrSta_enum] -> Equal40/1
  Relational Operator3/1 -> Terminator2/1  "VDDM_APSCorrErrDFS_flg"
  Equal40/1 -> Logical Operator37/2
  Constant59/1 -> DTC_Couter2/3
  Equal39/1 -> Logical Operator37/1
  DTC_Couter2/1 -> [VDDM_APSCorrErrCFS_flg]  "VDDM_APSCorrErrCFS_flg"
  [VDDM_APSCorrErrPass_flg] -> Logical Operator42/1
  [VDDM_APSCorrErrDet_flg] -> DTC_Couter2/1
  Logical Operator37/1 -> Logical Operator43/1
  Constant53/1 -> Logical Operator43/4
  Delay3/1 -> NOT3/1
  NOT3/1 -> Logical Operator42/2
  [DTC_clear_request] -> Logical Operator43/2
  Constant26/1 -> Equal40/2
  [VPMM_SysPwrSta_enum] -> Unit Delay4/1
  [VDDM_APSCorrErrCFSRls_flg] -> DTC_Couter2/2
  [VDDM_APS2SigOoRCFSRls_flg] -> Switch1/2
  [VDHP_EAPS2BAD_flg] -> Logical Operator13/1
  [VDDM_5vAPS2OoRCFS_flg] -> Logical Operator32/1
  Equal16/1 -> Logical Operator35/2
  Logical Operator32/1 -> Logical Operator35/3
  Constant50/1 -> DTC_Couter1/3
  [VDDM_APS2SigOoRDet_flg] -> DTC_Couter1/1
  Equal4/1 -> Logical Operator12/2
  Relational Operator1/1 -> Terminator1/1  "VDDM_APS2SigOoRDFS_flg"
  [VDDM_APS2SigOoRCFSRls_flg] -> DTC_Couter1/2
  [VDDM_APS2SigOoRPass_flg] -> Logical Operator29/1
  Logical Operator6/1 -> [VDDM_APS2SigOoRCFSRls_flg]  "VDDM_APS2SigOoRCFSRls_flg"
  Constant12/1 -> Logical Operator6/4
  Logical Operator12/1 -> Logical Operator6/1
  [VPMM_SysPwrSta_enum] -> Unit Delay3/1
  Constant11/1 -> Equal4/2
  [DTC_clear_request] -> Logical Operator6/2
  NOT2/1 -> Logical Operator29/2
  Delay2/1 -> NOT2/1
  DTC_Couter1/1 -> [VDDM_APS2SigOoRCFS_flg]  "VDDM_APS2SigOoRCFS_flg"
  Equal25/1 -> Logical Operator12/1
  Unit Delay3/1 -> Equal25/1
  Constant14/1 -> Equal25/2
  Constant13/1 -> Relational Operator1/2
  DTC_Couter1/2 -> Relational Operator1/1  "VDDM_APS2SigOoRDTC_cnt"
  Logical Operator29/1 -> Logical Operator6/3
  [VPMM_SysPwrSta_enum] -> Equal4/1
  [VDDM_APS2SigOoRCFS_flg] -> Delay2/1
  Logical Operator5/1 -> Switch1/3
  Logical Operator4/1 -> Logical Operator5/3
  Equal3/1 -> Logical Operator5/2
  [VDDM_5vAPS2OoRCFS_flg] -> Logical Operator4/1
  [VDHP_EAPS2BAD_flg] -> Logical Operator5/1
  Delay1/1 -> NOT1/1
  [VDDM_APS1SigOoRCFS_flg] -> Delay1/1
  Constant46/1 -> Logical Operator38/4
  [DTC_clear_request] -> Logical Operator38/2
  NOT1/1 -> Logical Operator41/2
  Constant45/1 -> Equal23/2
  Logical Operator39/1 -> Logical Operator38/1
  [VPMM_SysPwrSta_enum] -> Unit Delay6/1
  Relational Operator2/1 -> Terminator/1  "VDDM_APS1SigOoRDFS_flg"
  Equal23/1 -> Logical Operator39/2
  Constant48/1 -> Equal24/2
  Unit Delay6/1 -> Equal24/1
  [VPMM_SysPwrSta_enum] -> Equal23/1
  Equal24/1 -> Logical Operator39/1
  [VDDM_APS1SigOoRPass_flg] -> Logical Operator41/1
  Logical Operator41/1 -> Logical Operator38/3
  Constant49/1 -> DTC_Couter6/3
  DTC_Couter6/1 -> [VDDM_APS1SigOoRCFS_flg]  "VDDM_APS1SigOoRCFS_flg"
  Logical Operator38/1 -> [VDDM_APS1SigOoRCFSRls_flg]  "VDDM_APS1SigOoRCFSRls_flg"
  [VDDM_APS1SigOoRCFSRls_flg] -> DTC_Couter6/2
  DTC_Couter6/2 -> Relational Operator2/1  "VDDM_APS1SigOoRDTC_cnt"
  [VDDM_APS1SigOoRDet_flg] -> DTC_Couter6/1
  Constant47/1 -> Relational Operator2/2
  Logical Operator36/1 -> Logical Operator33/1
  [VDHP_EAPS1BAD_flg] -> Logical Operator36/1
  [VDDM_5vAPS1OoRCFS_flg] -> Logical Operator30/1
  Equal15/1 -> Logical Operator33/2
  Logical Operator30/1 -> Logical Operator33/3
  [VDDM_APSCorrErrPass_flg] -> DTC_Info2/2
  [VDDM_APSCorrErrDet_flg] -> DTC_Info2/1
  [VDDM_APS2SigOoRPass_flg] -> DTC_Info1/2
  [VDDM_APS2SigOoRDet_flg] -> DTC_Info1/1
  [VDDM_APS1SigOoRDet_flg] -> DTC_Info/1
  DTC_clear_request/1 -> [DTC_clear_request]
  task_time_s/1 -> [task_time_s]
  Logical Operator28/1 -> Logical Operator31/3
  Equal47/1 -> Logical Operator31/2
  [VDDM_5vAPS1OoRCFS_flg] -> Logical Operator28/1
  [VDHP_EAPS1BAD_flg] -> Logical Operator31/1
  Logical Operator73/1 -> Timer1/2
  Constant69/1 -> Equal28/2
  Timer1/1 -> Equal28/1
  Constant70/1 -> Timer1/4
  [task_time_s] -> Timer1/3
  Constant57/1 -> Test Detection Criteria1/4
  [task_time_s] -> Timer13/3
  Timer13/1 -> Equal55/1
  Logical Operator83/1 -> Timer13/2
  Test Detection Criteria1/1 -> [VDDM_APSCorrErrDet_flg]  "VDDM_APSCorrErrDet_flg"
  Constant91/1 -> Equal55/2
  [task_time_s] -> Test Detection Criteria1/2
  Constant55/1 -> Timer13/4
  Equal28/1 -> [VDDM_APS1SigOoRPass_flg]  "VDDM_APS1SigOoRPass_flg"
  Logical Operator35/1 -> Logical Operator112/1, Timer15/1
  Test Detection Criteria4/1 -> [VDDM_APS2SigOoRDet_flg]  "VDDM_APS2SigOoRDet_flg"
  Constant107/1 -> Equal65/2
  Constant108/1 -> Timer15/4
  Logical Operator112/1 -> Timer15/2
  Timer15/1 -> Equal65/1
  Equal65/1 -> [VDDM_APS2SigOoRPass_flg]  "VDDM_APS2SigOoRPass_flg"
  [task_time_s] -> Timer15/3
  Equal55/1 -> [VDDM_APSCorrErrPass_flg]  "VDDM_APSCorrErrPass_flg"
  Logical Operator49/1 -> Logical Operator83/1, Timer13/1
  [task_time_s] -> Test Detection Criteria3/2
  Constant86/1 -> Test Detection Criteria3/4
  Constant132/1 -> Test Detection Criteria3/3
  Test Detection Criteria3/1 -> [VDDM_APS1SigOoRDet_flg]  "VDDM_APS1SigOoRDet_flg"
  [VDDM_APS1SigOoRCFS_flg] -> DTC_Info/3
  [VDDM_APS1SigOoRPass_flg] -> DTC_Info/2
  DTC_Info/1 -> VDDM_APS1SigOoRDTC_raw32/1  "VDDM_APS1SigOoRDTC_raw32"
  Logical Operator33/1 -> Timer1/1, Logical Operator73/1
  [task_time_s] -> Test Detection Criteria4/2
  Constant15/1 -> Test Detection Criteria4/3
  Constant68/1 -> Test Detection Criteria4/4
  [VDDM_APS2SigOoRCFS_flg] -> DTC_Info1/3
  DTC_Info1/1 -> VDDM_APS2SigOoRDTC_raw32/1  "VDDM_APS2SigOoRDTC_raw32"
  VPMM_SysPwrSta_enum/1 -> [VPMM_SysPwrSta_enum]
  VINP_AccelPedal1Vol_V/1 -> [VINP_AccelPedal1Vol_V]
  VINP_AccelPedal2Vol_V/1 -> [VINP_AccelPedal2Vol_V]
  Constant58/1 -> Test Detection Criteria1/3
  [VDDM_APSCorrErrCFS_flg] -> DTC_Info2/3
  DTC_Info2/1 -> VDDM_APSCorrErrDTC_raw32/1  "VDDM_APSCorrErrDTC_raw32"
  VDHP_EAPS12RangeSta_enum/1 -> [VDHP_EAPS12RangeSta_enum]
  VDHP_EAPCRBAD_flg/1 -> [VDHP_EAPCRBAD_flg]
  [DTC_clear_request] -> DTC_Info/4
  [DTC_clear_request] -> DTC_Info1/4
  [DTC_clear_request] -> DTC_Info2/4
  [VDDM_APS1SigOoRCFSRls_flg] -> Switch6/2
  Switch6/1 -> Test Detection Criteria3/1
  Logical Operator31/1 -> Switch6/3
  Constant85/1 -> Switch6/1
  Switch1/1 -> Test Detection Criteria4/1
  Constant90/1 -> Switch1/1
  [VDDM_APSCorrErrCFSRls_flg] -> Switch2/2
  Switch2/1 -> Test Detection Criteria1/1
  Logical Operator86/1 -> Switch2/3
  Constant99/1 -> Switch2/1
  VINP_Pedal1Ref5V_V/1 -> [VINP_Pedal1Ref5V_V]
  VINP_Pedal2Ref5V_V/1 -> [VINP_Pedal2Ref5V_V]
  [VDDM_5vAPS1OoRCFS_flg] -> DTC_Info3/3
  [VDDM_5vAPS1OoRDet_flg] -> DTC_Info3/1
  Constant22/1 -> Test Detection Criteria2/4
  Timer4/1 -> Equal9/1
  Constant20/1 -> Timer4/4
  Logical Operator40/1 -> Timer4/2
  Test Detection Criteria2/1 -> [VDDM_5vAPS1OoRDet_flg]  "VDDM_5vAPS1OoRDet_flg"
  [VDDM_5vAPS1OoRCFSRls_flg] -> Switch3/2
  Constant19/1 -> Equal9/2
  [VDDM_5vAPS1OoRPass_flg] -> DTC_Info3/2
  Constant5/1 -> Test Detection Criteria2/3
  [task_time_s] -> Test Detection Criteria2/2
  [DTC_clear_request] -> DTC_Info3/4
  DTC_Info3/1 -> VDDM_5vAPS1OoRDTC_raw32/1  "VDDM_5vAPS1PwrErrDTC_raw32"
  Switch3/1 -> Test Detection Criteria2/1
  [task_time_s] -> Timer4/3
  Logical Operator7/1 -> Timer4/1, Logical Operator40/1
  Constant21/1 -> Switch3/1
  Equal9/1 -> [VDDM_5vAPS1OoRPass_flg]  "VDDM_5vAPS1OoRPass_flg"
  Equal2/1 -> Logical Operator2/1
  Equal5/1 -> Logical Operator2/2
  Logical Operator2/1 -> Logical Operator3/1
  Constant8/1 -> Equal2/2
  Constant9/1 -> Equal5/2
  Logical Operator3/1 -> Switch3/3
  [VINP_Pedal1Ref5V_V] -> Equal2/1
  [VINP_Pedal1Ref5V_V] -> Equal5/1
  VDHP_EAPS2BAD_flg/1 -> [VDHP_EAPS2BAD_flg]
  Switch4/1 -> Test Detection Criteria5/1
  [VDDM_5vAPS2OoRDet_flg] -> DTC_Info4/1
  Logical Operator22/1 -> Timer5/1, Logical Operator62/1
  Constant112/1 -> Test Detection Criteria5/4
  [VDDM_5vAPS2OoRCFSRls_flg] -> Switch4/2
  Constant30/1 -> Equal70/2
  [VDDM_5vAPS2OoRPass_flg] -> DTC_Info4/2
  [task_time_s] -> Test Detection Criteria5/2
  Constant118/1 -> Test Detection Criteria5/3
  [task_time_s] -> Timer5/3
  [DTC_clear_request] -> DTC_Info4/4
  Constant111/1 -> Switch4/1
  Constant109/1 -> Timer5/4
  [VDDM_5vAPS2OoRCFS_flg] -> DTC_Info4/3
  Equal70/1 -> [VDDM_5vAPS2OoRPass_flg]  "VDDM_5vAPS2OoRPass_flg"
  DTC_Info4/1 -> VDDM_5vAPS2OoRDTC_raw32/1  "VDDM_5vAPS2PwrErrDTC_raw32"
  Logical Operator62/1 -> Timer5/2
  Test Detection Criteria5/1 -> [VDDM_5vAPS2OoRDet_flg]  "VDDM_5vAPS2OoRDet_flg"
  Timer5/1 -> Equal70/1
  Logical Operator20/1 -> Switch4/3
  VDHP_EAPS1BAD_flg/1 -> [VDHP_EAPS1BAD_flg]
  Equal1/1 -> Logical Operator3/2
  [VINP_AccelPedal1Vol_V] -> Terminator5/1
  [VINP_AccelPedal2Vol_V] -> Terminator6/1
  [VDHP_EAPCRBAD_flg] -> Logical Operator86/2
  [VDHP_EAPCRBAD_flg] -> Logical Operator45/1
  Logical Operator45/1 -> Logical Operator49/2
